simulink model "lecture03g_model"  (R2021a)
settings: Solver=VariableStepAuto  StartTime=0.0  StopTime=tFinal_s  RelTol=1e-3
values from neighbouring files (symbols this model uses):
  A = [-2 1 ... (first row only)    [lecture03g.m]
  alpha = 2    [lecture03g.m]
  B = [3 -2 ... (first row only)    [lecture03g.m]
  C = eye(2)    [lecture03g.m]
  D = zeros(2,2)    [lecture03g.m]
  m = 20    [lecture03g.m]
  w = 10    [lecture03g.m]
  x0 = [3 ... (first row only)    [lecture03g.m]
libraries: simulink x1
settings Model: Creator=chris  LastModifiedBy=chris

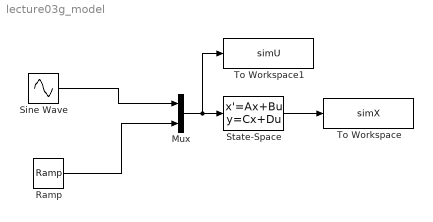
== system lecture03g_model ==
  Mux : Mux  Inputs=2
  Ramp : simulink/Sources/Ramp  slope=m  start=0  InitialOutput=0
  Sine Wave : Sin  Amplitude=alpha  Frequency=w  SampleTime=0
  State-Space : StateSpace  A=A  B=B  C=C  D=D  InitialCondition=x0
  To Workspace : ToWorkspace  VariableName=simX  SaveFormat=Timeseries  SampleTime=-1
  To Workspace1 : ToWorkspace  VariableName=simU  SaveFormat=Timeseries  SampleTime=-1
  wires:
  Sine Wave/1 -> Mux/1
  Ramp/1 -> Mux/2
  Mux/1 -> To Workspace1/1, State-Space/1
  State-Space/1 -> To Workspace/1
